simulink model "chap6_5sim"  (R2016a)
settings: Solver=VariableStepAuto  StartTime=0.0  StopTime=10.0  RelTol=1e-3
settings Model: Creator=zhanghankui  LastModifiedBy=zhanghankui

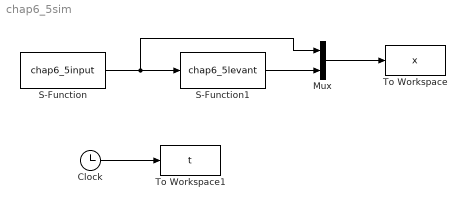
== system chap6_5sim ==
  Clock : Clock
  Mux : Mux  Inputs=2
  S-Function : S-Function  FunctionName=chap6_5input  SFunctionDeploymentMode=off  EnableBusSupport=off
  S-Function1 : S-Function  FunctionName=chap6_5levant  SFunctionDeploymentMode=off  EnableBusSupport=off
  To Workspace : ToWorkspace  VariableName=x  SampleTime=-1
  To Workspace1 : ToWorkspace  VariableName=t  SampleTime=-1
  wires:
  S-Function/1 -> Mux/1, S-Function1/1
  S-Function1/1 -> Mux/2
  Mux/1 -> To Workspace/1
  Clock/1 -> To Workspace1/1
